simulink model "Satellite_Attitude_Model"  (R2018b)
settings: Solver=ode23tb  StartTime=0.0  StopTime=1000  FixedStep=0.001  RelTol=1e-4
values from neighbouring files (symbols this model uses):
  A = [A11, A12; A21, A22]    [Satellite_Attitude_Model_Parameters.m]
  ArgOfPerigee_init = deg2rad (TLE_degree(5))    [Satellite_Attitude_Model_Parameters.m]
  b = 10e-6    (= 1e-05)    [Satellite_Attitude_Model_Parameters.m]
  B = [B11,B12; B21,B22]    [Satellite_Attitude_Model_Parameters.m]
  D = 0    [Satellite_Attitude_Model_Parameters.m]
  eccentricity_init = TLE_degree(4)    [Satellite_Attitude_Model_Parameters.m]
  Hconf4 = [Hgyro;Hstr]    [Satellite_Attitude_Model_Parameters.m]
  inclination_init = deg2rad (TLE_degree(2))    [Satellite_Attitude_Model_Parameters.m]
  Km = 0.1    [Satellite_Attitude_Model_Parameters.m]
  Kt = 0.1    [Satellite_Attitude_Model_Parameters.m]
  L = 5.2e-3    (= 0.0052)    [Satellite_Attitude_Model_Parameters.m]
  MeanAnomaly_init = deg2rad (TLE_degree(6))    [Satellite_Attitude_Model_Parameters.m]
  meanMotion_init = meanMotion_init*2*pi/86400    [Satellite_Attitude_Model_Parameters.m]
  Q = 1e-10    [Satellite_Attitude_Model_Parameters.m]
  q_init = [0; 0; 0; 1]    [Satellite_Attitude_Model_Parameters.m]
  R = 2    [Satellite_Attitude_Model_Parameters.m]    (also in dynamicFunctions2.m = 7078000)
  RAAN_init = deg2rad (TLE_degree(3))    [Satellite_Attitude_Model_Parameters.m]
  Rconf4 = [diag(ones(3,1))*Rgyro zeros(3,4);         zeros(4,3) diag(ones(1,4))*Rstr]    [Satellite_Attitude_Model_Parameters.m]
  Rgyro = 1e-12    [Satellite_Attitude_Model_Parameters.m]
  Rstr = 1e-12    [Satellite_Attitude_Model_Parameters.m]
  rw_Inertia = 5e-4    (= 0.0005)    [Satellite_Attitude_Model_Parameters.m]
  RW_Mmax = 0.015    [Satellite_Attitude_Model_Parameters.m]
  rw_SensorToBody = [0 0.4741 0.4741 -0.9482;                   -0.9999 0.3333 0.3333 0.3333;                    0 -0.8165 0.8165 0 ]    [Satellite_Attitude_Model_Parameters.m]
  RW_wmax = 300    [Satellite_Attitude_Model_Parameters.m]
  satInertia = [Isx 0 0 ; 0 Isy 0 ; 0 0 Isz]    [Satellite_Attitude_Model_Parameters.m]    (also in dynamicFunctions2.m = diag([Isx Isy Isz]))
  semimajor_init = sqrt(mu_earth^(1/3)/meanMotion_init^(2/3))    [Satellite_Attitude_Model_Parameters.m]
  Ts = 0.01    [Satellite_Attitude_Model_Parameters.m]
  unit7 = ones(7,1)    [Satellite_Attitude_Model_Parameters.m]
  w_dot_init = [0;0;0]    [Satellite_Attitude_Model_Parameters.m]
  w_init = [0; 0; 0]    [Satellite_Attitude_Model_Parameters.m]
  wRW_init = [0;0;0;0]    [Satellite_Attitude_Model_Parameters.m]
undefined symbols (not defined in the file or in its folder): Continuous, Earth, Time, WGS84
libraries: simulink x14, simulink_extras x13, sharedtransform x8, aerolibutil x2, sharedTrackingLibrary x1, ctrlSharedLib x1, aerolibtransform2 x1, aerolibgravity2 x1
(part 3 of 3)

== matlab function Satellite_Attitude_Model/Orbit Propagator Model/Orbit Propagator Model with Kepler Parameters(ECI)/MATLAB Function1 ==
  data: RAAN input; ArgOfPerigee input; semimajor input; inclination input; eccentricity input; trueAnomaly input; R_ECI output; Rdot_ECI output; v_Orbit output; r_Orbit output
function [ R_ECI, Rdot_ECI, v_Orbit, r_Orbit ] = aei2RdR( RAAN, ArgOfPerigee, semimajor, inclination, eccentricity, trueAnomaly )
% Converts Keplerian elements to Cartesian Rectangular Coordinates
% according to Chobotov section 4.8 pp. 62-65

% INPUTS
% semimajor      : Semi major axis [m]
% eccentricity   : Eccentricity
% inclination    : Inclination [rad]
% RAAN           : Right Ascension of the Ascending Node [rad]
% ArgOfPerigee   : Argument of Perigee [rad]
% trueAnomaly    : True Anomaly [rad]
% 
% OUTPUTS
% R_eci  : Satellite position in ECI frame [m]
% dR_eci : Satellite velocity in ECI frame [m/sec]
Rdot_ECI = zeros(3,1);
R_ECI = zeros(3,1);
v_Orbit = zeros(3,1);
r_Orbit = zeros(3,1);

% Earth Gravitational Constant [ in m3/sec2 ]
mu_earth = 398600.4418e9;

% Semilatus Rectum [m]
p = semimajor*(1-eccentricity*eccentricity) ;

% Magnitude of position vector [m]
r= p/(1+eccentricity*cos(trueAnomaly));

% Transformation matrix given in Chobotov pg. 65
R       =  zeros(3,3);
R(3,3)  =  cos(inclination);
R(3,2)  =  cos(ArgOfPerigee)*sin(inclination);
R(3,1)  =  sin(ArgOfPerigee)*sin(inclination);
R(2,3)  = -cos(RAAN)*sin(inclination);
R(2,2)  = -sin(RAAN)*sin(ArgOfPerigee) + cos(RAAN)*cos(ArgOfPerigee)*cos(inclination);
R(2,1)  =  sin(RAAN)*cos(ArgOfPerigee) + cos(RAAN)*sin(ArgOfPerigee)*cos(inclination);
R(1,3)  =  sin(RAAN)*sin(inclination);
R(1,2)  = -cos(RAAN)*sin(ArgOfPerigee) - sin(RAAN)*cos(ArgOfPerigee)*cos(inclination);
R(1,1)  =  cos(RAAN)*cos(ArgOfPerigee) - sin(RAAN)*sin(ArgOfPerigee)*cos(inclination);

% Position vector in ECI Frame[m]
R_ECI   = R * [  r*cos(trueAnomaly);
                 r*sin(trueAnomaly);
                 0          ];
             
             
% Velocity vector in ECI Frame [m/sec]
Rdot_ECI= R * [ -sqrt(mu_earth/p)*sin(trueAnomaly)     ;
                 sqrt(mu_earth/p)*(eccentricity+cos(trueAnomaly)) ;
                 0                       ];

% Velocity vector in Orbit Frame [m/sec]
vx = -sqrt(mu_earth/p)*sin(trueAnomaly);
vy = sqrt(mu_earth/p)*(eccentricity+ cos(trueAnomaly));
vz = zeros(1,size(trueAnomaly,2));

v_Orbit = [vx;vy;vz];

             
% Position vector in Orbit Frame [m/sec]
x = r*cos(trueAnomaly); 
y = r*sin(trueAnomaly);
z = zeros(1,size(trueAnomaly,2));

r_Orbit = [x;y;z];

end

== matlab function Satellite_Attitude_Model/Orbit Propagator Model/Orbit Propagator Model with Kepler Parameters(ECI)/Mean Anomaly To True Anomaly Transformation Model ==
  data: M input; trueAnomaly output; eccentricity input
% function trueAnomaly   = MeAn2TrAn( meanAnomaly,eccentricity )
% 
% % INPUTS
% % meanAnomaly  = Mean Anomaly [rad]
% % eccentricity = eccentricity
% % OUTPUTS
% % trueAnomaly  = True Anomaly [rad]
% 
% % Kepler's equation E=M+ecc*sin(E) (formula given in Chobotov pg 41)
% 
% E    = meanAnomaly; % Initial value for the eccentric anomaly
% delE = 1;
% tol  = 1e-12;
% while abs(delE)>tol
%     fE      = E - eccentricity*sin(E) - meanAnomaly ;
%     fdE     = 1 - eccentricity*cos(E);
%     delE    = -(fE/fdE);
%     E       = E + delE ;
% end
% 
% % Given Eccentric Anomaly to solve for True Anomaly (formula given in Chobotov pg 39)
% stht = (sqrt(1-eccentricity^2)*sin(E))/(1-eccentricity*cos(E));
% ctht = (cos(E)-eccentricity)/(1-eccentricity*cos(E));
% trueAnomaly = atan2(stht,ctht);
% 
% end

function trueAnomaly = findE(M,eccentricity)

% Tolerance = 1% 
tol   = 0.005;

% Error in E
err   = ones(1,size(M,2));

% Initial guess for E
E_old = ones(1,size(M,2)).*pi;
E_new = ones(1,size(M,2)).*pi;
while max(err) > tol
     
    % Find f(E)
    fE     = E_old - eccentricity*sin(E_old) - M;
    
    % Find f'(E)
    fE_derivative = 1 - eccentricity.*cos(E_old);
    
    % Find delta E
    dE     = fE./fE_derivative;

    % Calculate new E
    E_new  = E_old - dE;

    % Calculate % error in E
    err    = abs(E_new-E_old)./abs(E_old);
    
    % Update old value for E
    E_old  = E_new;
    
end

% Return E
E = E_new;

% Given Eccentric Anomaly to solve for True Anomaly (formula given in Chobotov pg 39)
stht = (sqrt(1-eccentricity^2)*sin(E))/(1-eccentricity*cos(E));
ctht = (cos(E)-eccentricity)/(1-eccentricity*cos(E));
trueAnomaly = atan2(stht,ctht);

end

== matlab function Satellite_Attitude_Model/Orbit Propagator Model/True Anomaly to Mean Anomaly/True Anomaly to Mean Anomaly ==
  data: ecc input; M output; TrAn input
function M   = TrAn2MeAn(ecc, TrAn )
% GIVEN TRUE ANOMALY, SOLVE FOR MEAN ANOMALY
% INPUTS
% TrAn = True Anomaly [rad]
% ecc = eccentricity
% OUTPUTS
% M   = Mean Anomaly [rad]

% Given True Anomaly, solve for Eccentric Anomaly 
% (formula given in Chobotov pg 37)
sE   = (sqrt(1-ecc^2)*sin(TrAn))/(1+ecc*cos(TrAn));
cE   = (cos(TrAn)+ecc)/(1+ecc*cos(TrAn));
E    = atan2(sE,cE);
% Calculate Mean Anomaly from Eccentric Anomaly
M    = E - ecc*sin(E);

== matlab function Satellite_Attitude_Model/Subsystem2/MATLAB Function ==
  data: q input; y output; p input
function y = qMult(q, p)

y=[p(4,1) p(3,1) -p(2,1) p(1,1);...
  -p(3,1) p(4,1) p(1,1) p(2,1);...
  p(2,1) -p(1,1) p(4,1) p(3,1);...
  -p(1,1) -p(2,1) -p(3,1) p(4,1)]*[q(1,1); q(2,1); q(3,1); q(4,1)];
end

== matlab function Satellite_Attitude_Model/Sun Position Model/Subsystem1/Sun Vector Model /SunVectorModel ==
  data: JD2000 input; sunVectorECI output; rECI input
function sunVectorECI = SunVectorModel( JD2000, rECI)

%   Sun Vector Model in Satellite Body Frame
%   References: The 1993 Astronomical Almanac, p. C24. 
% ----------------------------------------------------
%   INPUTS
% ----------------------------------------------------
%   JD2000   = (1x1) Julian Date 2000
%   rECI        = (3x1) Satellite Vector in ECI Frame [km]
%   qECI       = (4x1) Satellite Quaternion in ECI Frame
% 
%   PARAMETERS
% ----------------------------------------------------
%   distance = (1x1) Distance From Origin To Sun [km]
%
%   OUTPUTS
% ----------------------------------------------------
%   sunVectorBody   = (3x1) Unit Sun Vector 
% ----------------------------------------------------


% Degrees to Radians
% degToRad = pi / 180;

% Days From JD2000
days = JD2000 - 2451545.0;

% Mean Anomaly 
MeanAn = 357.528 + 0.9856003 * days;

% Ecliptic Longitude (lam)
lam  = rem( 280.460 + 0.9856474 * days, 360) + 1.915 * sind(MeanAn) + 0.02 * sind( 2 * MeanAn);

% Obliquity of Ecliptic
eclipticObliquity  = 23.439 - (4.00e-7 * days);

% Equatorial Rectangular Coordinates of Sun 
sLam = sind(lam);

sunVectorECI = [cosd(lam); cosd(eclipticObliquity).*sLam; sind(eclipticObliquity).*sLam];
distance = (1.0014 - 0.01671*cosd(MeanAn) - 0.00014*cosd(2*MeanAn))*149600e3;

% Account for parallax
sunVectorECI = [distance.*sunVectorECI(1,:) - rECI(1,:);...
                          distance.*sunVectorECI(2,:) - rECI(2,:);...
                          distance.*sunVectorECI(3,:) - rECI(3,:)];

                 
% Unit Sun Vector in ECI Frame
sunVectorECI = sunVectorECI / sqrt( sunVectorECI(1)*sunVectorECI(1) + sunVectorECI(2)*sunVectorECI(2) + sunVectorECI(3)*sunVectorECI(3));

== matlab function Satellite_Attitude_Model/Satellite Kinematic & Dynamic Model/Kinematic Model1/MATLAB Function ==
  data: w_OB_B input; y output
function y = skew_wOB_B(w_OB_B)


y = [0, w_OB_B(3,1), -w_OB_B(2,1), w_OB_B(1,1);...
    -w_OB_B(3,1), 0, w_OB_B(1,1), w_OB_B(2,1);...
     w_OB_B(2,1), -w_OB_B(1,1), 0, w_OB_B(3,1);...
    -w_OB_B(1,1), -w_OB_B(2,1), -w_OB_B(3,1), 0];
end

== matlab function Satellite_Attitude_Model/Subsystem2/MATLAB Function2 ==
  data: q_DCM output; r_ECI input; v_ECI input
function q_DCM  = LVLH2ECI( r_ECI, v_ECI)
%#codegen
%--------------------------------------------------------------------------
%   LVLH to ECI from q and w. Final angle is from ECI to ==> body. 
%--------------------------------------------------------------------------
%   Form:
%   [qEci, wBody] = LVLH2ECI(eulLVLH, wLVLH, rEci, vEci)
%--------------------------------------------------------------------------
%
%   ------
%   Inputs
%   ------
%   r               (3,1)   ECI position
%   v               (3,1)   ECI velocity
%   eulLVLH         (3,1)   RPY Euler angles in LVLH (rad)
%   wLVLH           (3,1)   Angular velocities in LVLH (rad/s)
%
%   -------
%   Outputs
%   -------
%   qEci2Body       (4,1)   ECI quaternion
%   wBody           (3,1)   Angular ve. in body frame(rad/s)
%
%--------------------------------------------------------------------------

% eci => lvlh
%-------------
q_DCM = QLVLH( r_ECI, v_ECI );

% eci => body
%------------

end

function DCM = QLVLH( r_ECI, v_ECI )
%   Generate the quaternions that transform from ECI to LVLH coordinates.

% LVLH Equations
y       = ( cross( v_ECI, r_ECI ) );
z       = ( -r_ECI );
x       = ( cross( y, z ) );

% x       =  r_ECI / norm(r_ECI);
% z       = (cross( r_ECI, v_ECI ))/norm(cross( r_ECI, v_ECI ));
% y       = (cross(z,x));


x = x/norm(x);
y = y/norm(y);
z = z/norm(z);

% Create DCM
DCM = [x'; y'; z'];

end

== matlab function Satellite_Attitude_Model/Satellite Kinematic & Dynamic Model/Kinematic Model1/Normalizer ==
  data: qnormalized output; q input
function qnormalized = fcn(q)

%Normalizes the quaternion

qnormalized = q;
qs = q(4);
qv = [q(1); q(2); q(3)];

qnormalized(4)= qs /norm(q);
qnormalized(1)= qv(1)/norm(q);
qnormalized(2)= qv(2)/norm(q);
qnormalized(3)= qv(3)/norm(q);

== matlab function Satellite_Attitude_Model/Satellite Kinematic & Dynamic Model/Kinematic Model1/MATLAB Function1 ==
  data: w_IB_B input; y output
function y = skew_wIB_B(w_IB_B)


y = [0, w_IB_B(3,1), -w_IB_B(2,1), w_IB_B(1,1);...
    -w_IB_B(3,1), 0, w_IB_B(1,1), w_IB_B(2,1);...
     w_IB_B(2,1), -w_IB_B(1,1), 0, w_IB_B(3,1);...
    -w_IB_B(1,1), -w_IB_B(2,1), -w_IB_B(3,1), 0];
end

== matlab function Satellite_Attitude_Model/Orbit Propagator Model/Orbit Propagator Model with Kepler Parameters(ECI)/Mean Motion To Semi-major Axis/MATLAB Function ==
  data: n input; semiMajor output
function semiMajor = meanMotionToSemimajor(n)
mu_earth = 398600.4418e9;
semiMajor = (mu_earth^(1/3))/(n^(2/3)); % meter
end

== matlab function Satellite_Attitude_Model/Orbit Propagator Model/Mean Motion To Semi-major Axis/MATLAB Function ==
  data: a input; meanMotion output
function meanMotion = semiMajorToMeanMotion(a)
mu_earth = 398600.4418e9;% meter
meanMotion = sqrt(mu_earth/a^3);
end

== matlab function Satellite_Attitude_Model/Actuator Model (RW)/Reaction Wheel Model ==
  data: rw_SensorToBody input; Hrw_dot_des output; inv_rwSensorToBody input; Mc input; w_IB_B input; wRw input
function Hrw_dot_des = rwModel(rw_SensorToBody,inv_rwSensorToBody,Mc,w_IB_B,wRw)
% The desired torque is calculated for each reaction wheel 

% The required momentum input
% wRw               (4x1) matrix
% rwInertia_matrix  (4x4) matrix
% rw_SensorToBody   (3x4) matrix
rwInertia = 5e-4; % RW moment of inertia (kg-m2)
rwInertia_matrix = eye(4,4)* rwInertia;
Hrw = rwInertia_matrix * wRw; 

% Hrw_B     (3x1) matrix
% Hrw_B_dot (3x1) matrix
% From Actuator Frame to Satellite Body Frame
Hrw_B = rw_SensorToBody * Hrw ;

% Desired reaction wheel torque in Body Frame
Hrw_B_dot = -Mc - cross(w_IB_B,Hrw_B) ;

% Desired reaction wheel torque in Actuator Frame
Hrw_dot_des = inv_rwSensorToBody * Hrw_B_dot ; 

end

== matlab function Satellite_Attitude_Model/MATLAB Function ==
  data: qref input; qerr_xyz output; qest input
function qerr_xyz  = quaternionError(qref, qest)

qerr = [qest(4)  qest(3) -qest(2) qest(1);...
       -qest(3)  qest(4)  qest(1) qest(2);...
        qest(2) -qest(1)  qest(4) qest(3);...
       -qest(1) -qest(2) -qest(3) qest(4)]*[-qref(1);-qref(2);-qref(3);qref(4)];

qerr_xyz = [qerr(1,1); qerr(2,1); qerr(3,1)];     
% qerr_x = qerr(1,1);
% qerr_y = qerr(2,1);
% qerr_z = qerr(3,1);

end
% % 
% function qerr_xyz  = quaternionError(qref, qest)
% 
% qerr = [qref(4)  -qref(3) qref(2) qref(1);...
%         qref(3)  qref(4)  -qref(1) qref(2);...
%         -qref(2) qref(1)  qref(4) qref(3);...
%        -qref(1) -qref(2) -qref(3) qref(4)]*[-qest(1);-qest(2);-qest(3);qest(4)];
% 
% qerr_xyz = [qerr(1,1); qerr(2,1); qerr(3,1)];     
% % qerr_x = qerr(1,1);
% % qerr_y = qerr(2,1);
% % qerr_z = qerr(3,1);
% 
% end

== matlab function Satellite_Attitude_Model/Total Disturbance Torque Model/Gravity Gradient Disturbance Torque Model/Last Column  ==
  data: DCM input; LastColumn_DCM output
function LastColumn_DCM = LastColumn(DCM)

LastColumn_DCM = zeros(3,1);
LastColumn_DCM(1,1) = DCM(1,3);
LastColumn_DCM(2,1) = DCM(2,3);
LastColumn_DCM(3,1) = DCM(3,3);

== matlab function Satellite_Attitude_Model/Total Disturbance Torque Model/Gravity Gradient Disturbance Torque Model/Skew Symmetric Matrix ==
  data: LastColumn_DCM input; SkewSym_DCM output
function SkewSym_DCM = SkewSym(LastColumn_DCM)

% LastColumn_DCM = [DCM(1,3); DCM(2,3); DCM(3,3)];
% LastColumn_DCM(1,1) = DCM(1,3)
% LastColumn_DCM(2,1) = DCM(2,3)
% LastColumn_DCM(3,1) = DCM(3,3)

SkewSym_DCM = [0 -LastColumn_DCM(3,1) LastColumn_DCM(2,1);...
                                LastColumn_DCM(3,1) 0 -LastColumn_DCM(1,1);...
                                 - LastColumn_DCM(2,1) LastColumn_DCM(1,1)  0];

== matlab function Satellite_Attitude_Model/Sensor Measurement Model (GYRO + STR)/Normalization Model/MATLAB Function ==
  data: u input; y output
function y = Sqrt(u)
%#codegen

y = sqrt(u);
